simulink model "massa_molla_smorzatore"  (R2019b)
settings: Solver=ode45  StartTime=par.sym.TStart  StopTime=par.sym.TStop  MaxStep=par.sym.max_dt  RelTol=1e-3  EnableMultiTasking=on
undefined symbols (not defined in the file): B, b, K, k, m, par, w_wav
settings Model: Creator=Vitù  LastModifiedBy=User
settings DataIOCC: SaveFormat=Array  SaveOutput=off  SignalLogging=off  DSMLogging=off  ReturnWorkspaceOutputs=off  TimeSaveName=TIME  OutputSaveName=Yout  OutputOption=AdditionalOutputTimes  OutputTimes=[par.sym.TStart:par.sym.Outputdt:par.sym.TStop]
settings OptimizationCC: ExpressionDepthLimit=2147483647  LifeSpan=inf
settings DebuggingCC: UnderspecifiedInitializationDetection=Classic  MergeDetectMultiDrivingBlocksExec=none  SolverPrmCheckMsg=warning  AllowSymbolicDim=off  StateNameClashWarn=warning  SFUnexpectedBacktrackingDiag=warning  SFNoUnconditionalDefaultTransitionDiag=warning  SFExecutionAtInitializationDiag=none  ArithmeticOperatorsInVariantConditions=warning
settings HardwareCC: ProdBitPerPointer=32  ProdBitPerSizeT=32  ProdBitPerPtrDiffT=32  ProdLargestAtomicFloat=None  ProdIntDivRoundTo=Undefined  ProdEndianess=Unspecified  ProdWordSize=32  ProdHWDeviceType=32-bit Generic
settings ModelReferenceCC: PropagateSignalLabelsOutOfModel=off
settings SFSimCC: SimUseLocalCustomCode=off  CustomCodeUndefinedFunction=UseInterfaceOnly
settings RTWCC: RTWUseLocalCustomCode=off
settings CodeAppCC: StateflowObjectComments=on
settings GRTTargetCC: TargetLangStandard=C89/C90 (ANSI)  GeneratePreprocessorConditionals=Disable all
settings ConfigComp: CovMetricSettings=dw  CovHtmlReporting=on  CovSaveCumulativeToWorkspaceVar=on  CovSaveSingleToWorkspaceVar=on  CovExternalEMLEnable=off  CovSFcnEnable=off
settings SimscapeCC: SimscapeNormalizeSystem=off
settings ConfigurationSet: Description=SimMechanics 2G

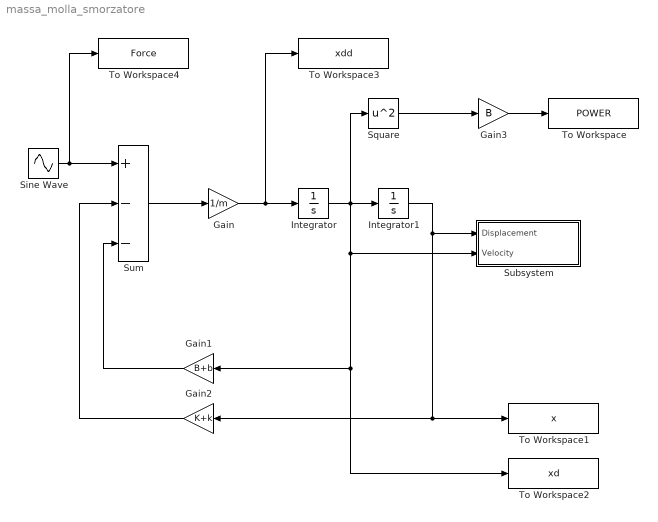
== system massa_molla_smorzatore ==
  Gain : Gain  Gain=1/m
  Gain1 : Gain  Gain=B+b
  Gain2 : Gain  Gain=K+k
  Gain3 : Gain  Gain=B
  Integrator : Integrator
  Integrator1 : Integrator
  Sine Wave : Sin  Amplitude=par.H  Frequency=w_wav  SampleTime=0
  Square : Math  Operator=square  SignedPower=off  SaturateOnIntegerOverflow=on
  Subsystem : Subsystem
  Sum : Sum  Inputs=+--
  To Workspace : ToWorkspace  VariableName=POWER  SampleTime=-1
  To Workspace1 : ToWorkspace  VariableName=x  SampleTime=-1
  To Workspace2 : ToWorkspace  VariableName=xd  SampleTime=-1
  To Workspace3 : ToWorkspace  VariableName=xdd  SampleTime=-1
  To Workspace4 : ToWorkspace  VariableName=Force  SampleTime=-1
  wires:
  Integrator1/1 -> Subsystem/1(Displacement), To Workspace1/1, Gain2/1
  Gain3/1 -> To Workspace/1
  Gain1/1 -> Sum/3
  Gain/1 -> To Workspace3/1, Integrator/1
  Square/1 -> Gain3/1
  Sum/1 -> Gain/1
  Integrator/1 -> Square/1, Subsystem/2(Velocity), To Workspace2/1, Gain1/1, Integrator1/1
  Gain2/1 -> Sum/2
  Sine Wave/1 -> To Workspace4/1, Sum/1

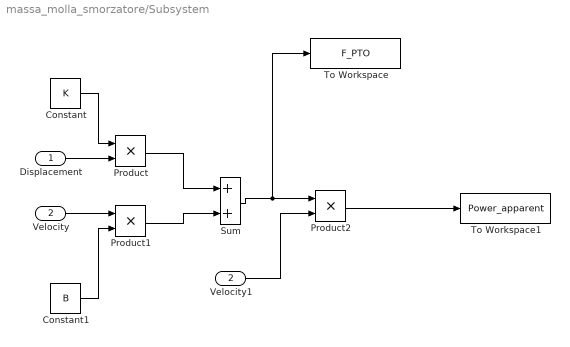
== system massa_molla_smorzatore/Subsystem ==
  Displacement : Inport
  Velocity : Inport  Port=2
  Constant : Constant  Value=K
  Constant1 : Constant  Value=B
  Product : Product
  Product1 : Product
  Product2 : Product
  Sum : Sum
  To Workspace : ToWorkspace  VariableName=F_PTO  SampleTime=-1
  To Workspace1 : ToWorkspace  VariableName=Power_apparent  SampleTime=-1
  Velocity1 : InportShadow  Port=2
  wires:
  Velocity/1 -> Product1/1
  Displacement/1 -> Product/2
  Constant/1 -> Product/1
  Constant1/1 -> Product1/2
  Product/1 -> Sum/1
  Product1/1 -> Sum/2
  Sum/1 -> To Workspace/1, Product2/1
  Velocity1/1 -> Product2/2
  Product2/1 -> To Workspace1/1
